simulink model "KalmanFilter"  (R2021a)
settings: Solver=VariableStepAuto  StartTime=0.0  StopTime=200  RelTol=1e-3
undefined symbols (not defined in the file or in its folder): A, Ad, B, Bd, Continuous, R, Time
libraries: simulink x1, ctrlSharedLib x1
settings Model: Creator=Panok  LastModifiedBy=Panok

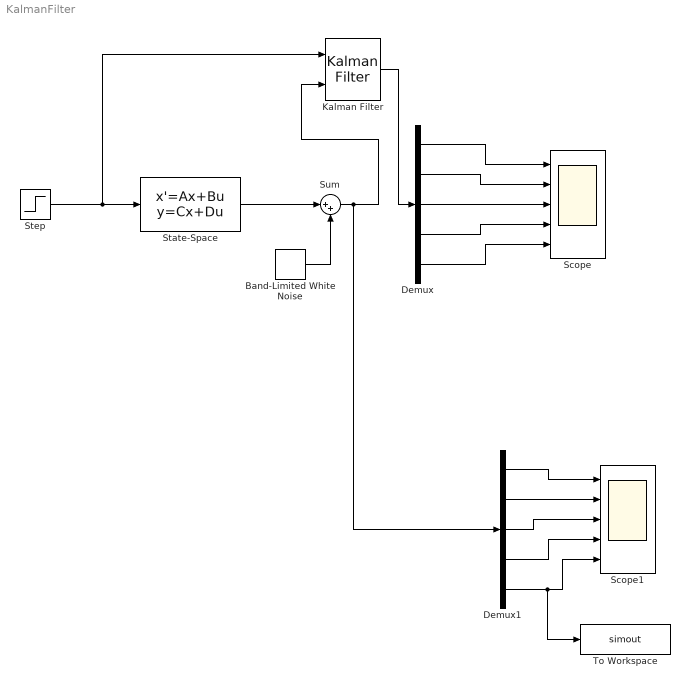
== system KalmanFilter ==
  Band-Limited White Noise : simulink/Sources/Band-Limited White Noise  Cov=[0.001; 0.000001; 0.000001; 0.000001; 0.001]  Ts=0.1  seed=[23341]
  Demux : Demux  Outputs=5
  Demux1 : Demux  Outputs=5
  Kalman Filter : ctrlSharedLib/Kalman Filter  TimeDomain=Continuous-Time  UseCurrentEstimator=on  ModelSource=Individual A, B, C, D matrices  ModelSourceVariable=ss(0.95,1,1,0,1)  A=Ad  B=Bd  C=eye(5)  D=0  NumberOfStates=1  NumberOfInputs=1  NumberOfOutputs=1  InitialEstimateSource=Dialog  X0=0  P0=10  UseK=off  UseGH=off  NumberOfProcessNoiseInputs=1  G=1  TimeInvariantG=on  H=0  TimeInvariantH=on  Q=0  TimeInvariantQ=on  R=R  TimeInvariantR=on  N=0  TimeInvariantN=on  AddInputPort=on  AddEnablePort=off  OutputEstimatedY=off  OutputP=off  Ts=-1
  Scope : Scope  NumInputPorts=5
  Scope1 : Scope  NumInputPorts=5
  State-Space : StateSpace  A=A  B=B  C=eye(5)  D=[0; 0; 0; 0; 0]  InitialCondition=0
  Step : Step  Time=0  After=-0.1  SampleTime=0
  Sum : Sum  Inputs=|++
  To Workspace : ToWorkspace  VariableName=simout  SaveFormat=Timeseries  SampleTime=-1
  wires:
  Step/1 -> Kalman Filter/1, State-Space/1
  Demux/1 -> Scope/1
  Demux/3 -> Scope/3
  Demux/2 -> Scope/2
  Demux/4 -> Scope/4
  Demux/5 -> Scope/5
  State-Space/1 -> Sum/1
  Kalman Filter/1 -> Demux/1
  Demux1/5 -> To Workspace/1, Scope1/5
  Sum/1 -> Demux1/1, Kalman Filter/2
  Demux1/1 -> Scope1/1
  Demux1/4 -> Scope1/4
  Demux1/2 -> Scope1/2
  Demux1/3 -> Scope1/3
  Band-Limited White Noise/1 -> Sum/2
